simulink model "part1"  (R2022a)
settings: Solver=VariableStepAuto  StartTime=0.0  StopTime=10.0  RelTol=1e-3
settings Model: Creator=21sao5  LastModifiedBy=21sao5

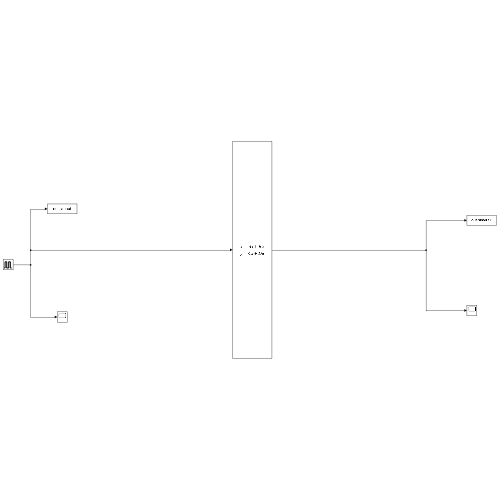
[thumbnail: Simulink's stored preview of the top-level diagram]
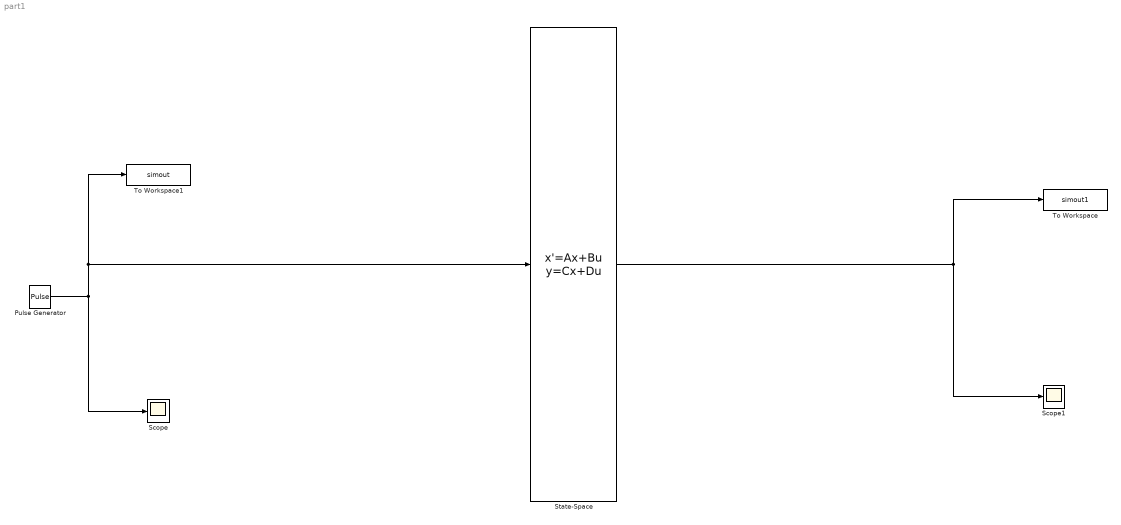
== system part1 ==
  Pulse Generator : DiscretePulseGenerator  PulseType=Time based  Amplitude=5  Period=10  PulseWidth=0.2/10*100
  Scope : Scope
  Scope1 : Scope
  State-Space : StateSpace  A=[0 1; 0 -35]  B=[0 ;200]  C=[1 0; 0 1]  D=[0; 0]  InitialCondition=0
  To Workspace : ToWorkspace  VariableName=simout1  SampleTime=-1
      settings: Save2DSignal=2-D array (concatenate along first dimension)
  To Workspace1 : ToWorkspace  VariableName=simout  SampleTime=-1
      settings: Save2DSignal=2-D array (concatenate along first dimension)
  wires:
  State-Space/1 -> To Workspace/1, Scope1/1
  Pulse Generator/1 -> To Workspace1/1, State-Space/1, Scope/1
